simulink model "PID_miniHopper_4_Pitch_Roll_Yaw_Contour_4"  (R2022b)
settings: Solver=VariableStepAuto  StartTime=0.0  StopTime=10  RelTol=1e-3
values from neighbouring files (symbols this model uses):
  hopper_ode = struct()    [MiniHopperParameters.m]
undefined symbols (not defined in the file or in its folder): A_rpy, B_rpy, Gain_pitch_U, Gain_roll_U, Gain_yaw_U, kT, VxLoop, VyLoop, XIC_rpy, XLoop, YLoop
libraries: simulink_extras x16, slpidlib x10
(part 2 of 2)

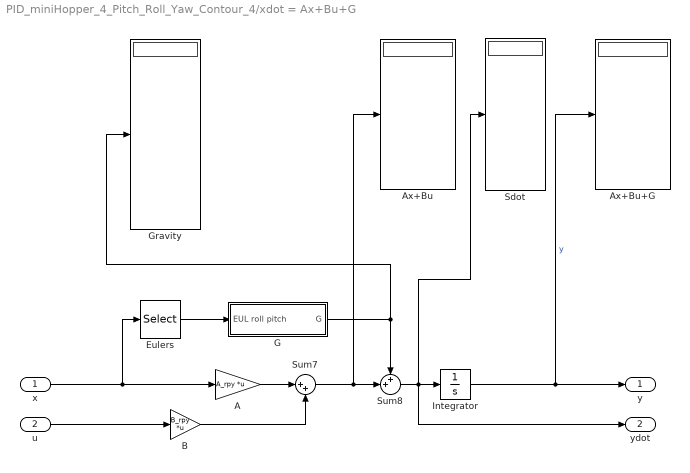
== system PID_miniHopper_4_Pitch_Roll_Yaw_Contour_4/xdot = Ax+Bu+G ==
  x : Inport
  u : Inport  Port=2
  A : Gain  Gain=A_rpy  Multiplication=Matrix(K*u)
  Ax+Bu : Display
  Ax+Bu+G : Display
  B : Gain  Gain=B_rpy  Multiplication=Matrix(K*u)
  Eulers : Selector  InputPortWidth=10  IndexOptions=Index vector (dialog)  Indices=[5 6 7]  OutputSizes=1
  G : Subsystem
  Gravity : Display
  Integrator : Integrator  InitialCondition=XIC_rpy
  Sdot : Display
  Sum7 : Sum  Inputs=|++
  Sum8 : Sum  Inputs=++|
  y : Outport
  ydot : Outport  Port=2
  wires:
  u/1 -> B/1
  B/1 -> Sum7/2
  Sum7/1 -> Ax+Bu/1, Sum8/2
  A/1 -> Sum7/1
  G/1(G) -> Gravity/1, Sum8/1
  x/1 -> Eulers/1, A/1
  Integrator/1 -> Ax+Bu+G/1, y/1  "y"
  Eulers/1 -> G/1(EUL roll pitch)
  Sum8/1 -> Sdot/1, ydot/1, Integrator/1

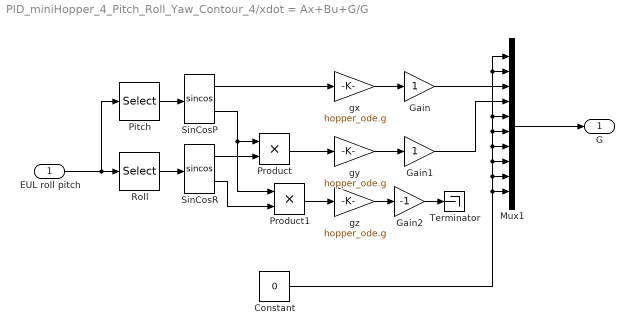
== system PID_miniHopper_4_Pitch_Roll_Yaw_Contour_4/xdot = Ax+Bu+G/G ==
  EUL roll pitch : Inport
  Constant : Constant  Value=0
  Gain : Gain
  Gain1 : Gain
  Gain2 : Gain  Gain=-1
  Mux1 : Mux  Inputs=10
  Pitch : Selector  InputPortWidth=3  IndexOptions=Index vector (dialog)  Indices=[2]  OutputSizes=1
  Product : Product
  Product1 : Product
  Roll : Selector  InputPortWidth=3  IndexOptions=Index vector (dialog)  Indices=[1]  OutputSizes=1
  SinCosP : Trigonometry  Operator=sincos
  SinCosR : Trigonometry  Operator=sincos
  Terminator : Terminator
  gx : Gain  Gain=hopper_ode.g
  gy : Gain  Gain=hopper_ode.g
  gz : Gain  Gain=hopper_ode.g
  G : Outport
  wires:
  Gain/1 -> Mux1/3
  Mux1/1 -> G/1
  Roll/1 -> SinCosR/1
  EUL roll pitch/1 -> Pitch/1, Roll/1
  SinCosP/2 -> Product1/1, Product/1
  SinCosR/1 -> Product/2
  gx/1 -> Gain/1
  Pitch/1 -> SinCosP/1
  SinCosP/1 -> gx/1
  Product/1 -> gy/1
  gy/1 -> Gain1/1
  Gain1/1 -> Mux1/4
  SinCosR/2 -> Product1/2
  Product1/1 -> gz/1
  gz/1 -> Gain2/1
  Gain2/1 -> Terminator/1
  Constant/1 -> Mux1/2, Mux1/1, Mux1/5, Mux1/6, Mux1/7, Mux1/8, Mux1/9, Mux1/10
